simulink model "raspberry_pi_send_video"  (R2016b)
settings: Solver=FixedStepAuto  StartTime=0.0  StopTime=10.0  RelTol=1e-3
libraries: embdlinuxlib x16, visionconversions x3
settings Model: SimulationMode=external  Creator=zeabus  LastModifiedBy=zeabus
settings SolverCC: PositivePriorityOrder=on
settings OptimizationCC: MaxStackSize=64
settings DebuggingCC: ParameterTunabilityLossMsg=error
settings HardwareCC: ProdBitPerPointer=32  ProdBitPerSizeT=32  ProdBitPerPtrDiffT=32  ProdLargestAtomicInteger=Long  ProdLargestAtomicFloat=Double  ProdWordSize=32  ProdHWDeviceType=ARM Compatible->ARM Cortex  UseEmbeddedCoderFeatures=off
settings RTWCC: SystemTargetFile=ert.tlc  HardwareBoard=Raspberry Pi  TLCOptions="-aInlineSetEventsForThisBaseRateFcn=TLC_FALSE -aSuppressMultiTaskScheduler=TLC_FALSE  -aRateBasedStepFcn=0"  TemplateMakefile=ert_default_tmf  Description=Embedded Coder  GenerateReport=on  Toolchain=GNU GCC Raspberry Pi  LaunchReport=on
settings CodeAppCC: ForceParamTrailComments=on  OperatorAnnotations=on  MATLABSourceComments=on
settings ERTTargetCC: ERTCustomFileBanners=off  SupportContinuousTime=on  SupportNonInlinedSFcns=on  RemoveResetFunc=off  SupportVariableSizeSignals=on  ModelStepFunctionPrototypeControlCompliant=off

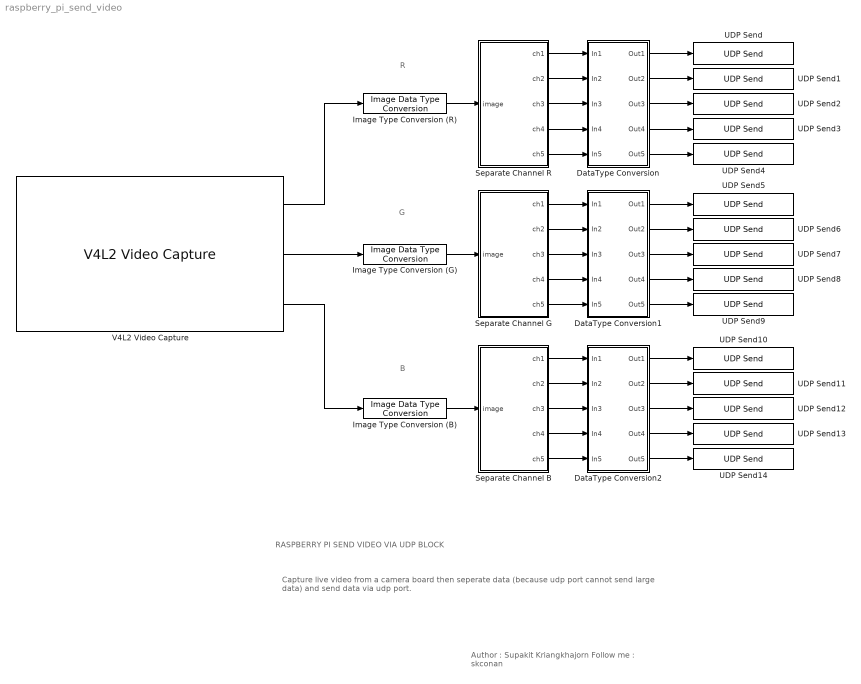
== system raspberry_pi_send_video ==
  note: R
  note: Capture live video from a camera board then seperate data (because udp port cannot send large data) and send data via udp port.
  note: Author : Supakit Kriangkhajorn
      | Follow me : skconan
  note: RASPBERRY PI SEND VIDEO VIA UDP BLOCK
  note: G
  note: B
  DataType Conversion : Subsystem
  DataType Conversion1 : Subsystem
  DataType Conversion2 : Subsystem
  "Image Type Conversion (B) " : visionconversions/Image Data Type Conversion  outDT=uint8  isSigned=on  wordLen=16  numFracBits=0
  "Image Type Conversion (G) " : visionconversions/Image Data Type Conversion  outDT=uint8  isSigned=on  wordLen=16  numFracBits=0
  "Image Type Conversion (R) " : visionconversions/Image Data Type Conversion  outDT=uint8  isSigned=on  wordLen=16  numFracBits=0
  Separate Channel B : MATLAB Function  TreatAsAtomicUnit=on
  Separate Channel G : MATLAB Function  TreatAsAtomicUnit=on
  Separate Channel R : MATLAB Function  TreatAsAtomicUnit=on
  UDP Send : embdlinuxlib/UDP Send  remoteURL='192.168.1.189'  remotePort=30000  localURL='255.255.255.255'  localPortSource=Automatically determine  localPort=-1  sampletime=-1  blockPlatform=Raspberry Pi  separateLengthPort=0
  UDP Send1 : embdlinuxlib/UDP Send  remoteURL='192.168.1.189'  remotePort=30001  localURL='255.255.255.255'  localPortSource=Automatically determine  localPort=-1  sampletime=-1  blockPlatform=Raspberry Pi  separateLengthPort=0
  UDP Send10 : embdlinuxlib/UDP Send  remoteURL='192.168.1.189'  remotePort=30010  localURL='255.255.255.255'  localPortSource=Automatically determine  localPort=-1  sampletime=-1  blockPlatform=Raspberry Pi  separateLengthPort=0
  UDP Send11 : embdlinuxlib/UDP Send  remoteURL='192.168.1.189'  remotePort=30011  localURL='255.255.255.255'  localPortSource=Automatically determine  localPort=-1  sampletime=-1  blockPlatform=Raspberry Pi  separateLengthPort=0
  UDP Send12 : embdlinuxlib/UDP Send  remoteURL='192.168.1.189'  remotePort=30012  localURL='255.255.255.255'  localPortSource=Automatically determine  localPort=-1  sampletime=-1  blockPlatform=Raspberry Pi  separateLengthPort=0
  UDP Send13 : embdlinuxlib/UDP Send  remoteURL='192.168.1.189'  remotePort=30013  localURL='255.255.255.255'  localPortSource=Automatically determine  localPort=-1  sampletime=-1  blockPlatform=Raspberry Pi  separateLengthPort=0
  UDP Send14 : embdlinuxlib/UDP Send  remoteURL='192.168.1.189'  remotePort=30014  localURL='255.255.255.255'  localPortSource=Automatically determine  localPort=-1  sampletime=-1  blockPlatform=Raspberry Pi  separateLengthPort=0
  UDP Send2 : embdlinuxlib/UDP Send  remoteURL='192.168.1.189'  remotePort=30002  localURL='255.255.255.255'  localPortSource=Automatically determine  localPort=-1  sampletime=-1  blockPlatform=Raspberry Pi  separateLengthPort=0
  UDP Send3 : embdlinuxlib/UDP Send  remoteURL='192.168.1.189'  remotePort=30003  localURL='255.255.255.255'  localPortSource=Automatically determine  localPort=-1  sampletime=-1  blockPlatform=Raspberry Pi  separateLengthPort=0
  UDP Send4 : embdlinuxlib/UDP Send  remoteURL='192.168.1.189'  remotePort=30004  localURL='255.255.255.255'  localPortSource=Automatically determine  localPort=-1  sampletime=-1  blockPlatform=Raspberry Pi  separateLengthPort=0
  UDP Send5 : embdlinuxlib/UDP Send  remoteURL='192.168.1.189'  remotePort=30005  localURL='255.255.255.255'  localPortSource=Automatically determine  localPort=-1  sampletime=-1  blockPlatform=Raspberry Pi  separateLengthPort=0
  UDP Send6 : embdlinuxlib/UDP Send  remoteURL='192.168.1.189'  remotePort=30006  localURL='255.255.255.255'  localPortSource=Automatically determine  localPort=-1  sampletime=-1  blockPlatform=Raspberry Pi  separateLengthPort=0
  UDP Send7 : embdlinuxlib/UDP Send  remoteURL='192.168.1.189'  remotePort=30007  localURL='255.255.255.255'  localPortSource=Automatically determine  localPort=-1  sampletime=-1  blockPlatform=Raspberry Pi  separateLengthPort=0
  UDP Send8 : embdlinuxlib/UDP Send  remoteURL='192.168.1.189'  remotePort=30008  localURL='255.255.255.255'  localPortSource=Automatically determine  localPort=-1  sampletime=-1  blockPlatform=Raspberry Pi  separateLengthPort=0
  UDP Send9 : embdlinuxlib/UDP Send  remoteURL='192.168.1.189'  remotePort=30009  localURL='255.255.255.255'  localPortSource=Automatically determine  localPort=-1  sampletime=-1  blockPlatform=Raspberry Pi  separateLengthPort=0
  V4L2 Video Capture : embdlinuxlib/V4L2 Video Capture  m_devName='/dev/video0'  roi=[0, 0, 640, 480]  imSizeSelection=320x240  imSize=[240, 320]  pixelFormat=RGB  pixelOrder=Planar  sampleTime=1/30  simOutput=Colorbars  blockPlatform=Raspberry Pi
  wires:
  V4L2 Video Capture/1 -> "Image Type Conversion (R) "/1
  V4L2 Video Capture/2 -> "Image Type Conversion (G) "/1
  V4L2 Video Capture/3 -> "Image Type Conversion (B) "/1
  "Image Type Conversion (R) "/1 -> Separate Channel R/1(image)
  "Image Type Conversion (G) "/1 -> Separate Channel G/1(image)
  "Image Type Conversion (B) "/1 -> Separate Channel B/1(image)
  Separate Channel B/1(ch1) -> DataType Conversion2/1(In1)
  Separate Channel B/2(ch2) -> DataType Conversion2/2(In2)
  Separate Channel B/4(ch4) -> DataType Conversion2/4(In4)
  Separate Channel B/3(ch3) -> DataType Conversion2/3(In3)
  Separate Channel B/5(ch5) -> DataType Conversion2/5(In5)
  Separate Channel R/1(ch1) -> DataType Conversion/1(In1)
  Separate Channel R/2(ch2) -> DataType Conversion/2(In2)
  Separate Channel R/3(ch3) -> DataType Conversion/3(In3)
  Separate Channel R/4(ch4) -> DataType Conversion/4(In4)
  Separate Channel R/5(ch5) -> DataType Conversion/5(In5)
  DataType Conversion/5(Out5) -> UDP Send4/1
  DataType Conversion/4(Out4) -> UDP Send3/1
  DataType Conversion/3(Out3) -> UDP Send2/1
  DataType Conversion/2(Out2) -> UDP Send1/1
  DataType Conversion/1(Out1) -> UDP Send/1
  Separate Channel G/1(ch1) -> DataType Conversion1/1(In1)
  Separate Channel G/2(ch2) -> DataType Conversion1/2(In2)
  Separate Channel G/3(ch3) -> DataType Conversion1/3(In3)
  Separate Channel G/4(ch4) -> DataType Conversion1/4(In4)
  Separate Channel G/5(ch5) -> DataType Conversion1/5(In5)
  DataType Conversion1/5(Out5) -> UDP Send9/1
  DataType Conversion1/4(Out4) -> UDP Send8/1
  DataType Conversion1/3(Out3) -> UDP Send7/1
  DataType Conversion1/2(Out2) -> UDP Send6/1
  DataType Conversion1/1(Out1) -> UDP Send5/1
  DataType Conversion2/1(Out1) -> UDP Send10/1
  DataType Conversion2/2(Out2) -> UDP Send11/1
  DataType Conversion2/3(Out3) -> UDP Send12/1
  DataType Conversion2/4(Out4) -> UDP Send13/1
  DataType Conversion2/5(Out5) -> UDP Send14/1

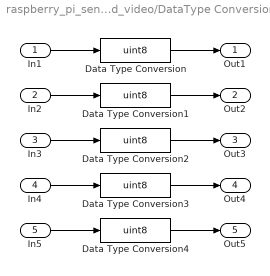
== system raspberry_pi_send_video/DataType Conversion ==
  In1 : Inport
  In2 : Inport  Port=2
  In3 : Inport  Port=3
  In4 : Inport  Port=4
  In5 : Inport  Port=5
  Data Type Conversion{,1..4} (5 alike) : DataTypeConversion  OutDataTypeStr=uint8
  Out1 : Outport
  Out2 : Outport  Port=2
  Out3 : Outport  Port=3
  Out4 : Outport  Port=4
  Out5 : Outport  Port=5
  wires:
  In1/1 -> Data Type Conversion/1
  In2/1 -> Data Type Conversion1/1
  In4/1 -> Data Type Conversion3/1
  In3/1 -> Data Type Conversion2/1
  In5/1 -> Data Type Conversion4/1
  Data Type Conversion/1 -> Out1/1
  Data Type Conversion1/1 -> Out2/1
  Data Type Conversion2/1 -> Out3/1
  Data Type Conversion3/1 -> Out4/1
  Data Type Conversion4/1 -> Out5/1

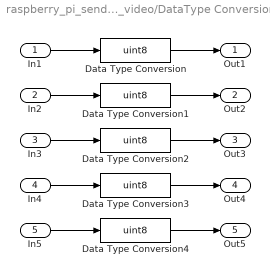
== system raspberry_pi_send_video/DataType Conversion1 ==
  In1 : Inport
  In2 : Inport  Port=2
  In3 : Inport  Port=3
  In4 : Inport  Port=4
  In5 : Inport  Port=5
  Data Type Conversion{,1..4} (5 alike) : DataTypeConversion  OutDataTypeStr=uint8
  Out1 : Outport
  Out2 : Outport  Port=2
  Out3 : Outport  Port=3
  Out4 : Outport  Port=4
  Out5 : Outport  Port=5
  wires:
  In1/1 -> Data Type Conversion/1
  In2/1 -> Data Type Conversion1/1
  In4/1 -> Data Type Conversion3/1
  In3/1 -> Data Type Conversion2/1
  In5/1 -> Data Type Conversion4/1
  Data Type Conversion/1 -> Out1/1
  Data Type Conversion1/1 -> Out2/1
  Data Type Conversion2/1 -> Out3/1
  Data Type Conversion3/1 -> Out4/1
  Data Type Conversion4/1 -> Out5/1

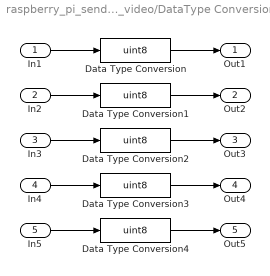
== system raspberry_pi_send_video/DataType Conversion2 ==
  In1 : Inport
  In2 : Inport  Port=2
  In3 : Inport  Port=3
  In4 : Inport  Port=4
  In5 : Inport  Port=5
  Data Type Conversion{,1..4} (5 alike) : DataTypeConversion  OutDataTypeStr=uint8
  Out1 : Outport
  Out2 : Outport  Port=2
  Out3 : Outport  Port=3
  Out4 : Outport  Port=4
  Out5 : Outport  Port=5
  wires:
  In1/1 -> Data Type Conversion/1
  In2/1 -> Data Type Conversion1/1
  In4/1 -> Data Type Conversion3/1
  In3/1 -> Data Type Conversion2/1
  In5/1 -> Data Type Conversion4/1
  Data Type Conversion/1 -> Out1/1
  Data Type Conversion1/1 -> Out2/1
  Data Type Conversion2/1 -> Out3/1
  Data Type Conversion3/1 -> Out4/1
  Data Type Conversion4/1 -> Out5/1

== matlab function raspberry_pi_send_video/Separate Channel G ==
  data: image input; ch1 output; ch2 output; ch3 output; ch4 output; ch5 output
function [ch1,ch2,ch3,ch4,ch5] = separate(image)
maxlength = 76800;
dividelength = 15360;

image = reshape(image,1,maxlength);
ch1 = image(1:dividelength);
ch2 = image(dividelength*1+1:dividelength*2);
ch3 = image(dividelength*2+1:dividelength*3);
ch4 = image(dividelength*3+1:dividelength*4);
ch5 = image(dividelength*4+1:dividelength*5);

== matlab function raspberry_pi_send_video/Separate Channel R ==
  data: image input; ch1 output; ch2 output; ch3 output; ch4 output; ch5 output
function [ch1,ch2,ch3,ch4,ch5] = separate(image)
maxlength = 76800;
dividelength = 15360;

image = reshape(image,1,maxlength);
ch1 = image(1:dividelength);
ch2 = image(dividelength*1+1:dividelength*2);
ch3 = image(dividelength*2+1:dividelength*3);
ch4 = image(dividelength*3+1:dividelength*4);
ch5 = image(dividelength*4+1:dividelength*5);

== matlab function raspberry_pi_send_video/Separate Channel B ==
  data: image input; ch1 output; ch2 output; ch3 output; ch4 output; ch5 output
function [ch1,ch2,ch3,ch4,ch5] = separate(image)
maxlength = 76800;
dividelength = 15360;

image = reshape(image,1,maxlength);
ch1 = image(1:dividelength);
ch2 = image(dividelength*1+1:dividelength*2);
ch3 = image(dividelength*2+1:dividelength*3);
ch4 = image(dividelength*3+1:dividelength*4);
ch5 = image(dividelength*4+1:dividelength*5);
